simulink model "sampleModel1936_5"  (R2023a)
settings: Solver=VariableStepAuto  StartTime=0.0  StopTime=10.0  RelTol=1e-3
libraries: hdlsllib x7
settings Model: Creator=user1  LastModifiedBy=user1

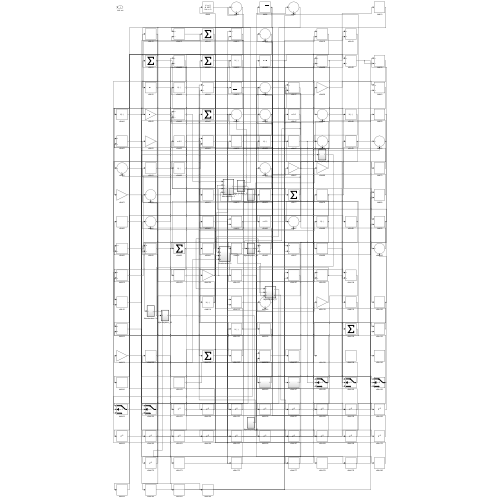
[thumbnail: Simulink's stored preview of the top-level diagram]
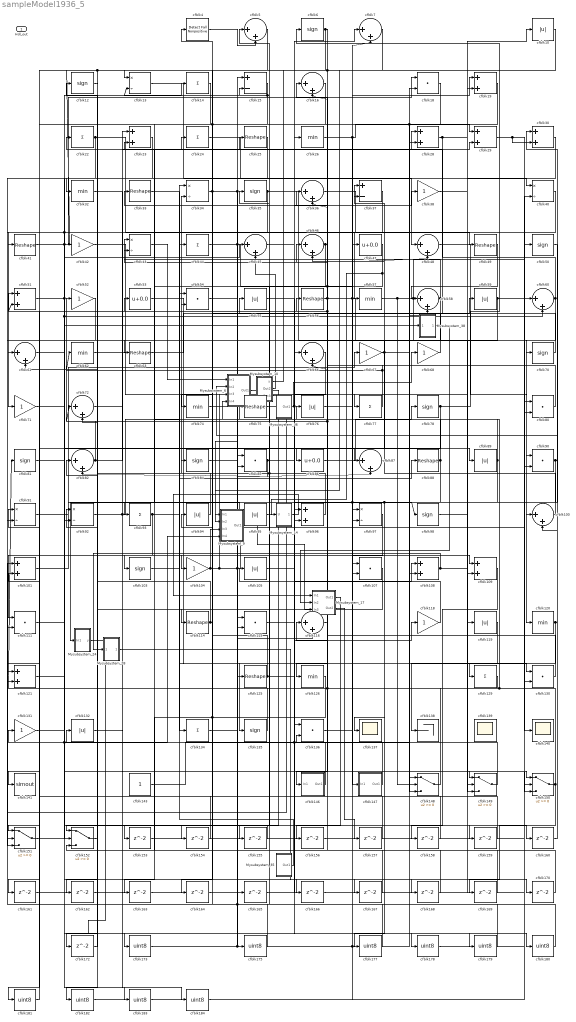
== system sampleModel1936_5 ==
  Mysubsystem_10 : Subsystem  TreatAsAtomicUnit=on  RTWFcnName=Mysubsystem_10
      settings: RTWFcnNameOpts=User specified  RTWFileNameOpts=Use function name
  Mysubsystem_14 : Subsystem  TreatAsAtomicUnit=on  RTWFcnName=Mysubsystem_14
      settings: RTWFcnNameOpts=User specified  RTWFileNameOpts=Use function name
  Mysubsystem_17 : Subsystem  TreatAsAtomicUnit=on  RTWFcnName=Mysubsystem_17
      settings: RTWFcnNameOpts=User specified  RTWFileNameOpts=Use function name
  Mysubsystem_24 : Subsystem  TreatAsAtomicUnit=on  RTWFcnName=Mysubsystem_24
      settings: RTWFcnNameOpts=User specified  RTWFileNameOpts=Use function name
  Mysubsystem_28 : Subsystem  TreatAsAtomicUnit=on  RTWFcnName=Mysubsystem_28
      settings: RTWFcnNameOpts=User specified  RTWFileNameOpts=Use function name
  Mysubsystem_35 : Subsystem  TreatAsAtomicUnit=on  RTWFcnName=Mysubsystem_35
      settings: RTWFcnNameOpts=User specified  RTWFileNameOpts=Use function name
  Mysubsystem_36 : Subsystem  TreatAsAtomicUnit=on  RTWFcnName=Mysubsystem_36
      settings: RTWFcnNameOpts=User specified  RTWFileNameOpts=Use function name
  Mysubsystem_38 : Subsystem  TreatAsAtomicUnit=on  RTWFcnName=Mysubsystem_38
      settings: RTWFcnNameOpts=User specified  RTWFileNameOpts=Use function name
  Mysubsystem_6 : Subsystem  TreatAsAtomicUnit=on  RTWFcnName=Mysubsystem_6
      settings: RTWFcnNameOpts=User specified  RTWFileNameOpts=Use function name
  Mysubsystem_9 : Subsystem  TreatAsAtomicUnit=on  RTWFcnName=Mysubsystem_9
      settings: RTWFcnNameOpts=User specified  RTWFileNameOpts=Use function name
  cfblk{10,55,59,76,89,94..95,105,119,132} (10 alike) : Abs  OutDataTypeStr=uint8  SaturateOnIntegerOverflow=off
  cfblk{5,7,16,36,45..46,48,58,60..61,66,72,82,87,100,116} (16 alike) : Sum  Inputs=|++  OutDataTypeStr=uint8
  cfblk{19,23,28..30,51,96,101,108..109,121} (11 alike) : Sum  OutDataTypeStr=uint8
  cfblk{6,12,35,50,70,78,81,84,98,103,135} (11 alike) : Signum
  cfblk{38,42,52,67..68,71,104,118,131} (9 alike) : Gain  OutDataTypeStr=uint8
  cfblk{18,54,80,85,90,107,111,115,130,136} (10 alike) : DotProduct  OutDataTypeStr=uint8
  cfblk{25,33,41,49,56,63,75,88,114,125} (10 alike) : Reshape
  cfblk{26,32,57,62,74,120,126} (7 alike) : MinMax  OutDataTypeStr=uint8
  cfblk{14,22,24,44,77,93,129,134} (8 alike) : Sum  Inputs=+  OutDataTypeStr=uint8
  cfblk{13,34,40,43,91..92,97} (7 alike) : Product  Inputs=*/  OutDataTypeStr=uint8  RndMeth=Zero  SaturateOnIntegerOverflow=on
  cfblk137 : Scope
  cfblk138 : Terminator
  cfblk139 : Scope
      settings: Floating=on
  cfblk140 : Scope
  cfblk141 : ToWorkspace  VariableName=simout  SaveFormat=Timeseries  SampleTime=-1
  cfblk143 : Constant  OutDataTypeStr=uint8  SampleTime=-1
  cfblk146 : Subsystem
      settings: LibrarySourceBlock=|
      | hdlsllib/Ports &
      | Subsystems/Subsystem
  cfblk147 : Subsystem
      settings: LibrarySourceBlock=|
      | hdlsllib/Ports &
      | Subsystems/Subsystem
  cfblk{148..152} (5 alike) : Switch  OutDataTypeStr=uint8  SaturateOnIntegerOverflow=off  InputSameDT=off
  cfblk15 : Sum  Inputs=+-  OutDataTypeStr=uint8
  cfblk{153..170,172} (19 alike) : Delay  SampleTime=1
  cfblk{173,175,177..184} (10 alike) : DataTypeConversion  OutDataTypeStr=uint8  SaturateOnIntegerOverflow=off  RndMeth=Floor
  cfblk37 : Sum  Inputs=+-  OutDataTypeStr=uint8
  cfblk4 : hdlsllib/Logic and Bit Operations/Detect Fall Nonpositive  vinit=0  OutDataTypeStr=uint8
  cfblk47 : Bias  Bias=0.0  SaturateOnIntegerOverflow=off
  cfblk53 : Bias  Bias=0.0  SaturateOnIntegerOverflow=off
  cfblk86 : Bias  Bias=0.0  SaturateOnIntegerOverflow=off
  Hdl_out : Outport  OutDataTypeStr=uint8
  wires:
  cfblk58/1 -> cfblk43/1, cfblk151/2
  cfblk74/1 -> cfblk77/1
  cfblk49/1 -> cfblk55/1
  cfblk78/1 -> cfblk6/1, cfblk141/1
  cfblk150/1 -> Mysubsystem_6/4(In4), cfblk81/1, cfblk36/1, cfblk169/1
  cfblk82/1 -> cfblk52/1, cfblk25/1
  cfblk97/1 -> cfblk103/1
  cfblk41/1 -> cfblk18/1, cfblk150/1
  cfblk101/1 -> cfblk67/1
  cfblk53/1 -> cfblk135/1
  cfblk88/1 -> Mysubsystem_24/1(In1), cfblk53/1
  cfblk108/1 -> Mysubsystem_28/1(In1), cfblk150/2
  cfblk70/1 -> cfblk4/1
  cfblk130/1 -> cfblk36/2, cfblk51/2, cfblk72/1
  cfblk13/1 -> cfblk97/1
  cfblk48/1 -> cfblk120/1
  cfblk94/1 -> cfblk34/2
  cfblk93/1 -> cfblk111/1, cfblk88/1
  cfblk5/1 -> cfblk121/1
  cfblk118/1 -> cfblk35/1
  cfblk63/1 -> cfblk59/1
  cfblk125/1 -> cfblk24/1, cfblk118/1
  cfblk26/1 -> cfblk29/1, cfblk48/2
  cfblk33/1 -> cfblk89/1
  cfblk126/1 -> cfblk163/1, cfblk164/1
  cfblk46/1 -> cfblk16/1, cfblk155/1
  cfblk35/1 -> cfblk92/2, cfblk111/2, cfblk148/1
  cfblk51/1 -> cfblk14/1, cfblk159/1
  cfblk56/1 -> cfblk90/1, cfblk7/2, cfblk16/2
  cfblk22/1 -> cfblk57/1, cfblk91/2
  cfblk15/1 -> cfblk13/2, cfblk181/1
  cfblk40/1 -> cfblk71/1
  cfblk96/1 -> cfblk15/2, cfblk61/2
  cfblk131/1 -> cfblk180/1
  cfblk76/1 -> cfblk109/1
  cfblk129/1 -> cfblk121/2
  cfblk6/1 -> cfblk126/1, cfblk13/1
  cfblk114/1 -> cfblk84/1, cfblk12/1
  cfblk148/1 -> cfblk76/1, cfblk51/1
  cfblk66/1 -> cfblk96/2
  cfblk34/1 -> cfblk29/2, cfblk87/2, cfblk154/1
  cfblk47/1 -> Mysubsystem_14/1(U), cfblk66/2, cfblk63/1
  cfblk68/1 -> cfblk5/1
  cfblk30/1 -> cfblk104/1
  cfblk147/1(Out1) -> cfblk136/2
  cfblk90/1 -> Mysubsystem_6/2(In2), cfblk177/1
  cfblk80/1 -> cfblk33/1
  cfblk98/1 -> cfblk109/2
  cfblk115/1 -> cfblk108/1
  cfblk24/1 -> cfblk48/1
  cfblk87/1 -> cfblk37/1
  cfblk59/1 -> cfblk60/1, cfblk87/1
  cfblk62/1 -> cfblk134/1
  cfblk28/1 -> cfblk10/1, cfblk58/1
  cfblk89/1 -> cfblk137/1, cfblk115/2, cfblk75/1
  cfblk135/1 -> cfblk82/1
  cfblk60/1 -> cfblk22/1, cfblk70/1
  cfblk95/1 -> cfblk149/1
  cfblk103/1 -> cfblk129/1
  cfblk50/1 -> cfblk100/1
  cfblk120/1 -> cfblk30/1, cfblk149/3
  cfblk71/1 -> cfblk85/2
  cfblk143/1 -> cfblk26/1, cfblk28/2
  cfblk119/1 -> cfblk138/1
  cfblk72/1 -> cfblk23/1
  cfblk23/1 -> cfblk152/2
  cfblk151/1 -> Mysubsystem_38/1(In1), Mysubsystem_9/4(In4)
  cfblk146/1(Out1) -> cfblk91/1
  cfblk29/1 -> cfblk140/1, cfblk30/2
  cfblk136/1 -> cfblk19/1
  cfblk45/1 -> cfblk7/1
  cfblk57/1 -> cfblk119/1, cfblk40/2, cfblk148/2
  cfblk37/1 -> cfblk146/1(In1)
  cfblk67/1 -> cfblk130/1, cfblk37/2
  cfblk84/1 -> cfblk116/2
  cfblk36/1 -> cfblk49/1
  cfblk100/1 -> cfblk46/2
  cfblk14/1 -> cfblk41/1
  cfblk19/1 -> cfblk114/1, cfblk151/1, cfblk108/2
  cfblk85/1 -> cfblk82/2, cfblk28/1
  cfblk44/1 -> Mysubsystem_9/2(In2), cfblk147/1(In1)
  cfblk91/1 -> cfblk95/1
  cfblk4/1 -> cfblk5/2
  cfblk111/1 -> cfblk45/1, cfblk60/2
  cfblk86/1 -> cfblk78/1
  cfblk75/1 -> cfblk98/1, cfblk97/2, cfblk38/1
  cfblk152/1 -> cfblk92/1
  cfblk18/1 -> cfblk61/1
  cfblk92/1 -> cfblk44/1, cfblk150/3
  cfblk38/1 -> cfblk40/1
  cfblk104/1 -> Mysubsystem_9/3(In3), Mysubsystem_6/3(In3), cfblk50/1, cfblk148/3
  cfblk77/1 -> cfblk62/1, cfblk43/2
  cfblk10/1 -> cfblk86/1, cfblk74/1
  cfblk116/1 -> cfblk56/1
  cfblk42/1 -> cfblk149/2
  cfblk16/1 -> cfblk93/1
  cfblk149/1 -> cfblk132/1
  cfblk153/1 -> cfblk90/2
  cfblk154/1 -> cfblk101/2
  cfblk155/1 -> cfblk152/1
  cfblk156/1 -> cfblk46/1
  cfblk157/1 -> cfblk34/1
  cfblk109/1 -> cfblk158/1
  cfblk158/1 -> cfblk15/1
  cfblk159/1 -> cfblk136/1
  cfblk121/1 -> cfblk160/1
  cfblk160/1 -> cfblk100/2
  cfblk52/1 -> cfblk161/1
  cfblk161/1 -> cfblk85/1
  cfblk25/1 -> cfblk162/1
  cfblk163/1 -> cfblk66/1
  cfblk164/1 -> cfblk130/2
  cfblk134/1 -> cfblk165/1
  cfblk165/1 -> cfblk19/2
  cfblk166/1 -> cfblk18/2
  cfblk81/1 -> cfblk167/1
  cfblk167/1 -> cfblk152/3
  cfblk55/1 -> cfblk168/1
  cfblk168/1 -> cfblk116/1
  cfblk169/1 -> cfblk23/2
  cfblk132/1 -> cfblk170/1
  cfblk170/1 -> cfblk96/1
  cfblk12/1 -> cfblk172/1
  cfblk172/1 -> cfblk72/2
  cfblk173/1 -> cfblk58/2, cfblk47/1, cfblk125/1
  cfblk54/1 -> cfblk175/1
  cfblk175/1 -> cfblk94/1
  cfblk177/1 -> cfblk54/2
  cfblk105/1 -> cfblk178/1
  cfblk178/1 -> cfblk80/2
  cfblk32/1 -> cfblk179/1
  cfblk179/1 -> cfblk105/1
  cfblk180/1 -> cfblk115/1, cfblk101/1
  cfblk181/1 -> cfblk131/1
  cfblk107/1 -> cfblk182/1
  cfblk182/1 -> cfblk80/1
  cfblk61/1 -> cfblk183/1
  cfblk183/1 -> cfblk107/1
  cfblk162/1 -> cfblk184/1
  cfblk184/1 -> cfblk107/2
  cfblk43/1 -> Mysubsystem_6/1(In1)
  Mysubsystem_6/1(Out1) -> cfblk153/1
  cfblk7/1 -> Mysubsystem_9/1(In1)
  Mysubsystem_10/1(y) -> cfblk42/1, cfblk32/1
  Mysubsystem_10/2(Out2) -> cfblk45/2
  Mysubsystem_10/3(Out3) -> cfblk151/3
  Mysubsystem_14/1(Out1) -> Mysubsystem_17/1(In1)
  Mysubsystem_9/1(Out1) -> Mysubsystem_17/3(In3)
  Mysubsystem_17/1(Out1) -> cfblk156/1
  Mysubsystem_17/2(Out2) -> cfblk157/1
  Mysubsystem_24/1(y) -> cfblk173/1
  Mysubsystem_28/1(Out1) -> cfblk166/1
  Mysubsystem_35/1(Out1) -> cfblk54/1
  Mysubsystem_36/1(Out1) -> cfblk68/1
  Mysubsystem_38/1(Out1) -> Mysubsystem_17/2(In2)

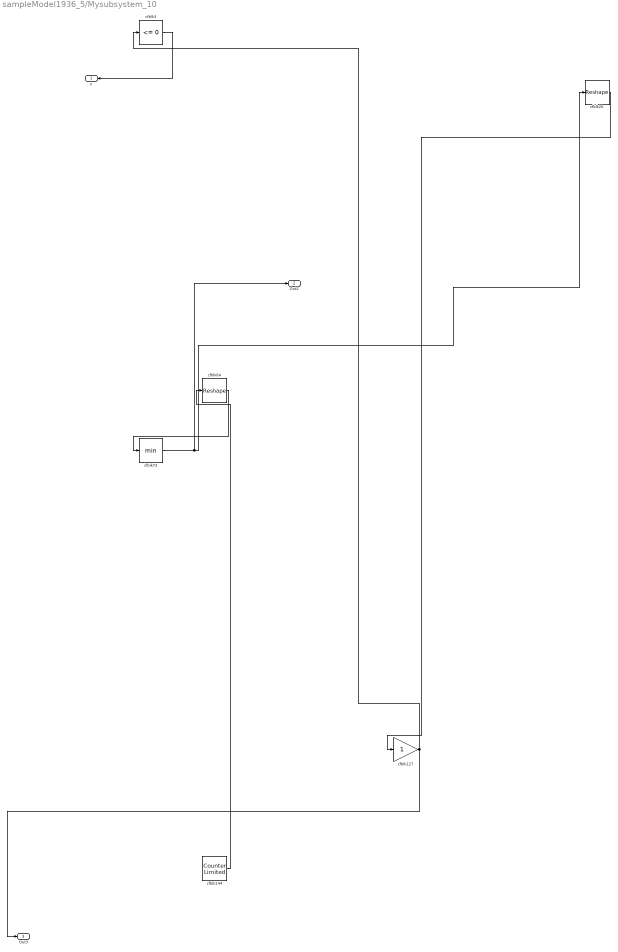
== system sampleModel1936_5/Mysubsystem_10 ==
  cfblk127 : Gain
  cfblk144 : hdlsllib/Sources/Counter Limited  uplimit=7  tsamp=-1
  cfblk20 : Reshape
  cfblk3 : hdlsllib/Logic and Bit Operations/Compare To Zero  relop=<=  OutDataTypeStr=boolean
  cfblk64 : Reshape
  cfblk73 : MinMax
  y : Outport
  Out2 : Outport  Port=2
  Out3 : Outport  Port=3
  wires:
  cfblk64/1 -> cfblk73/1
  cfblk3/1 -> y/1
  cfblk20/1 -> cfblk127/1
  cfblk144/1 -> cfblk64/1
  cfblk127/1 -> Out3/1, cfblk3/1
  cfblk73/1 -> Out2/1, cfblk20/1

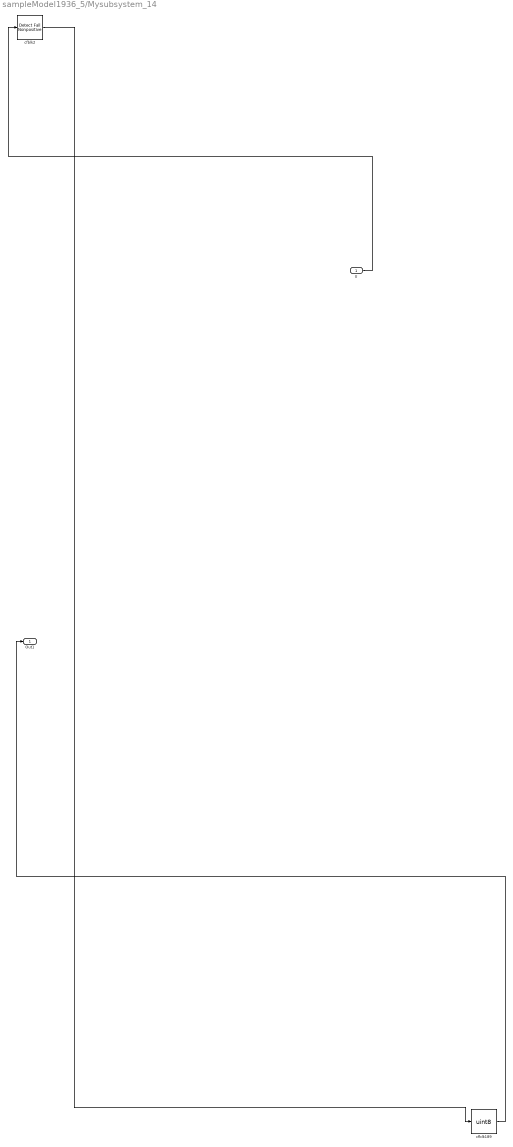
== system sampleModel1936_5/Mysubsystem_14 ==
  U : Inport
  cfblk189 : DataTypeConversion  OutDataTypeStr=uint8  SaturateOnIntegerOverflow=off  RndMeth=Floor
  cfblk2 : hdlsllib/Logic and Bit Operations/Detect Fall Nonpositive  vinit=0  OutDataTypeStr=boolean
  Out1 : Outport
  wires:
  U/1 -> cfblk2/1
  cfblk2/1 -> cfblk189/1
  cfblk189/1 -> Out1/1

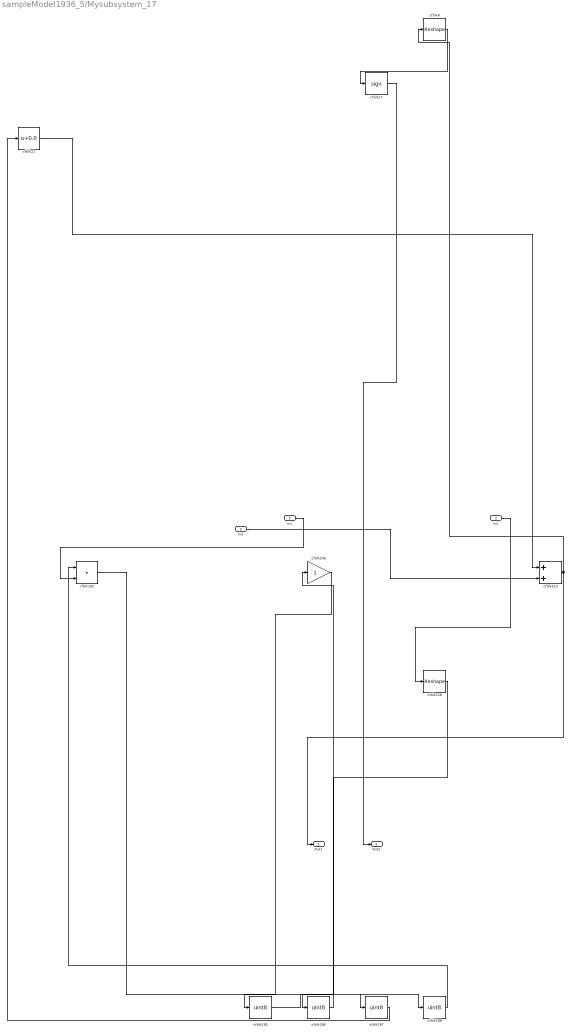
== system sampleModel1936_5/Mysubsystem_17 ==
  In1 : Inport
  In2 : Inport  Port=2
  In3 : Inport  Port=3
  cfblk102 : DotProduct  OutDataTypeStr=Inherit: Inherit via internal rule
  cfblk106 : Gain
  cfblk110 : Sum
  cfblk128 : Reshape
  cfblk17 : Signum
  cfblk{185..188} (4 alike) : DataTypeConversion  OutDataTypeStr=uint8  SaturateOnIntegerOverflow=off  RndMeth=Floor
  cfblk21 : Bias  Bias=0.0  SaturateOnIntegerOverflow=off
  cfblk8 : Reshape
  Out1 : Outport
  Out2 : Outport  Port=2
  wires:
  cfblk21/1 -> cfblk110/1
  cfblk128/1 -> cfblk186/1
  cfblk186/1 -> cfblk106/1
  cfblk187/1 -> cfblk21/1
  In3/1 -> cfblk110/2
  cfblk110/1 -> Out1/1, cfblk8/1
  cfblk185/1 -> cfblk188/1
  cfblk106/1 -> cfblk185/1
  cfblk188/1 -> cfblk102/1
  cfblk102/1 -> cfblk187/1
  cfblk8/1 -> cfblk17/1
  In2/1 -> cfblk128/1
  In1/1 -> cfblk102/2
  cfblk17/1 -> Out2/1

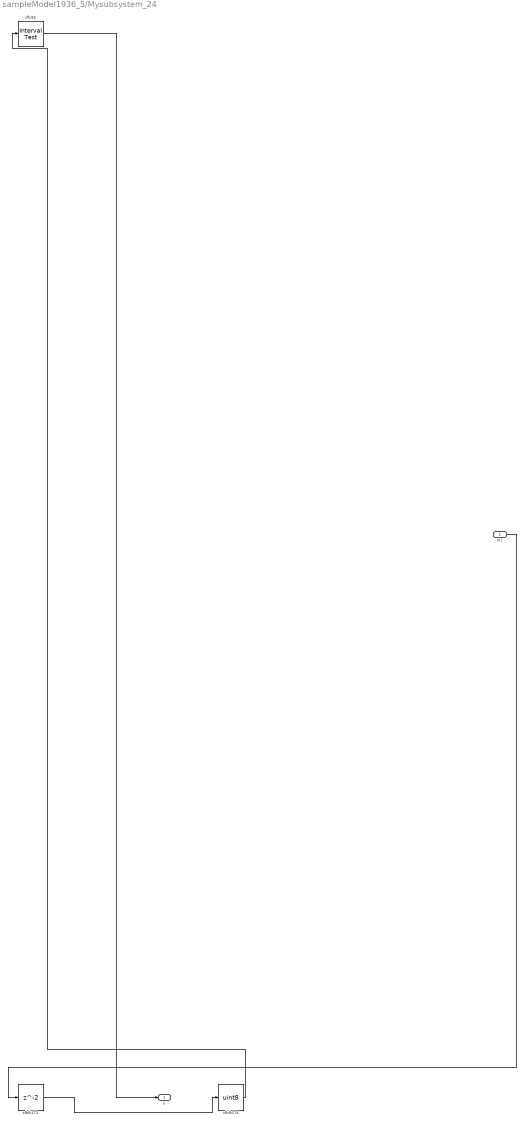
== system sampleModel1936_5/Mysubsystem_24 ==
  In1 : Inport
  cfblk1 : hdlsllib/Logic and Bit Operations/Interval Test  IntervalClosedRight=on  uplimit=0.5  IntervalClosedLeft=on  lowlimit=-0.5  OutDataTypeStr=boolean
  cfblk171 : Delay  SampleTime=1
  cfblk174 : DataTypeConversion  OutDataTypeStr=uint8  SaturateOnIntegerOverflow=off  RndMeth=Floor
  y : Outport
  wires:
  cfblk171/1 -> cfblk174/1
  cfblk174/1 -> cfblk1/1
  In1/1 -> cfblk171/1
  cfblk1/1 -> y/1

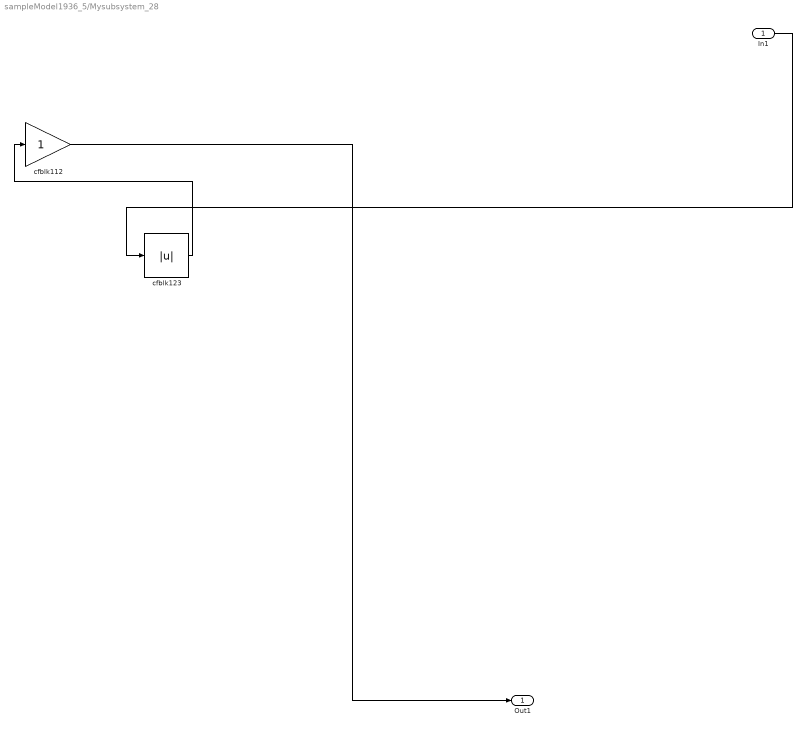
== system sampleModel1936_5/Mysubsystem_28 ==
  In1 : Inport
  cfblk112 : Gain
  cfblk123 : Abs  SaturateOnIntegerOverflow=off
  Out1 : Outport
  wires:
  cfblk123/1 -> cfblk112/1
  In1/1 -> cfblk123/1
  cfblk112/1 -> Out1/1

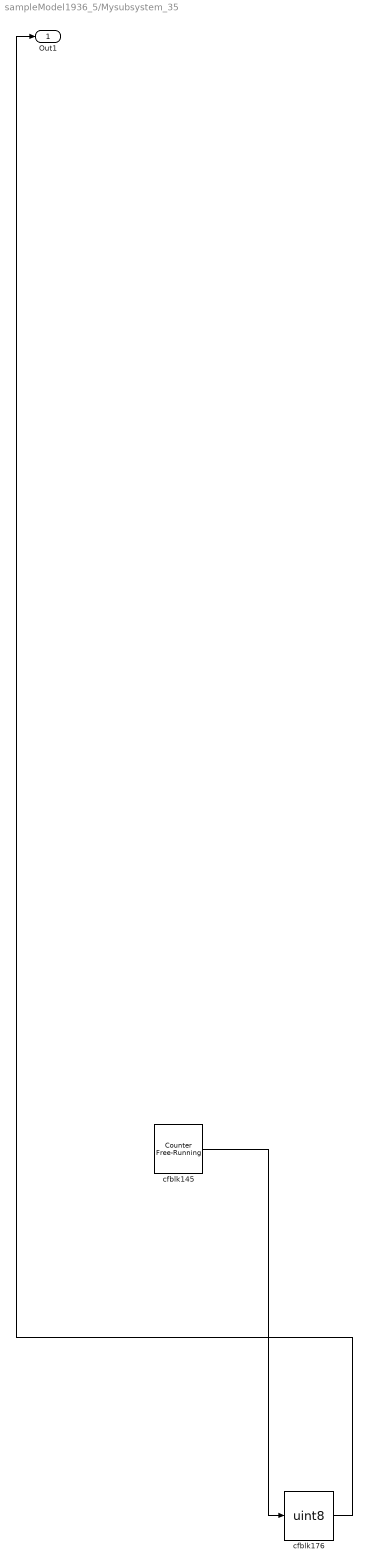
== system sampleModel1936_5/Mysubsystem_35 ==
  cfblk145 : hdlsllib/Sources/Counter Free-Running  NumBits=16  tsamp=-1
  cfblk176 : DataTypeConversion  OutDataTypeStr=uint8  SaturateOnIntegerOverflow=off  RndMeth=Floor
  Out1 : Outport
  wires:
  cfblk145/1 -> cfblk176/1
  cfblk176/1 -> Out1/1

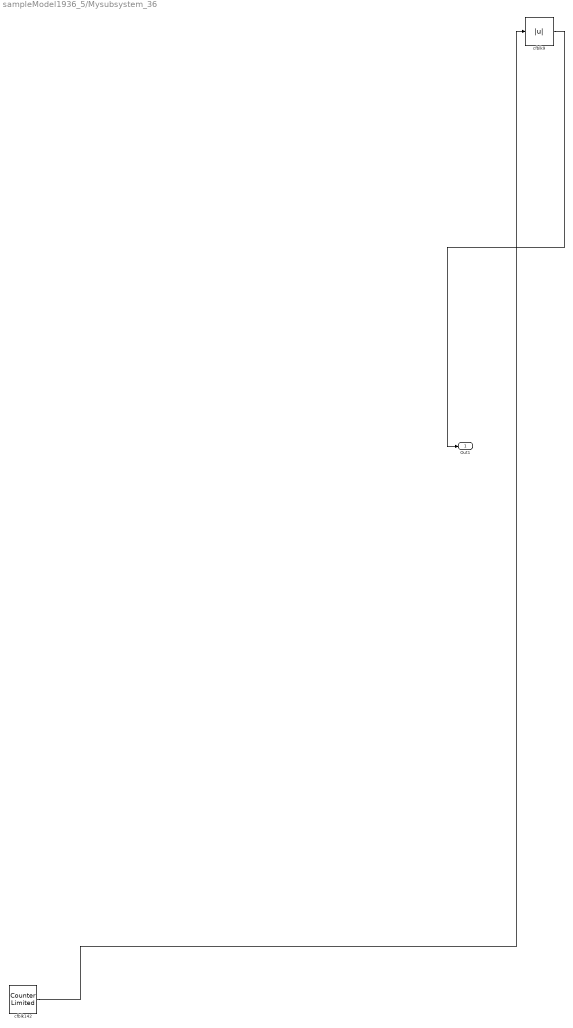
== system sampleModel1936_5/Mysubsystem_36 ==
  cfblk142 : hdlsllib/Sources/Counter Limited  uplimit=7  tsamp=-1
  cfblk9 : Abs  SaturateOnIntegerOverflow=off
  Out1 : Outport
  wires:
  cfblk142/1 -> cfblk9/1
  cfblk9/1 -> Out1/1

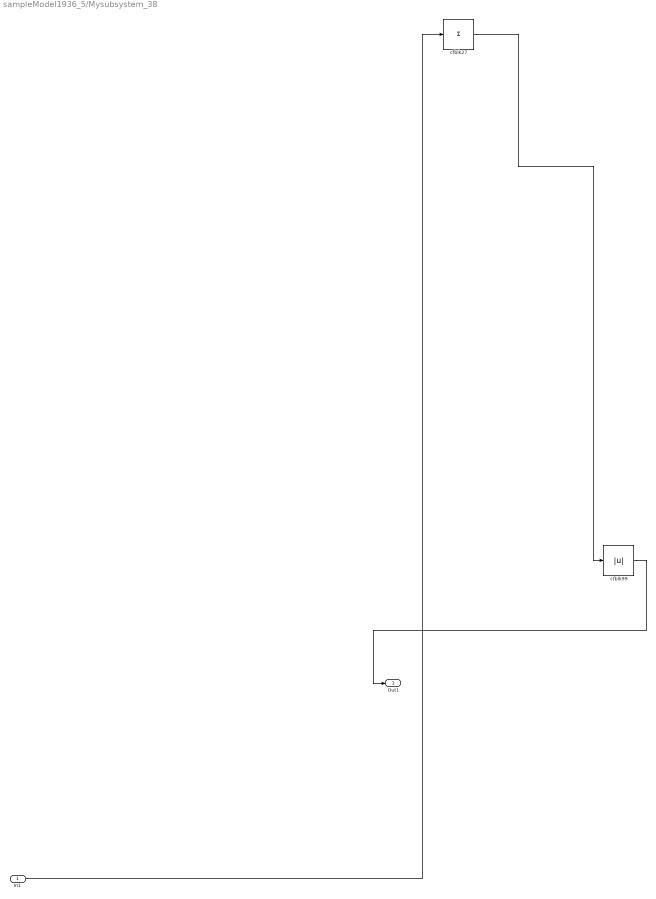
== system sampleModel1936_5/Mysubsystem_38 ==
  In1 : Inport
  cfblk27 : Sum  Inputs=+
  cfblk99 : Abs  SaturateOnIntegerOverflow=off
  Out1 : Outport
  wires:
  cfblk27/1 -> cfblk99/1
  cfblk99/1 -> Out1/1
  In1/1 -> cfblk27/1

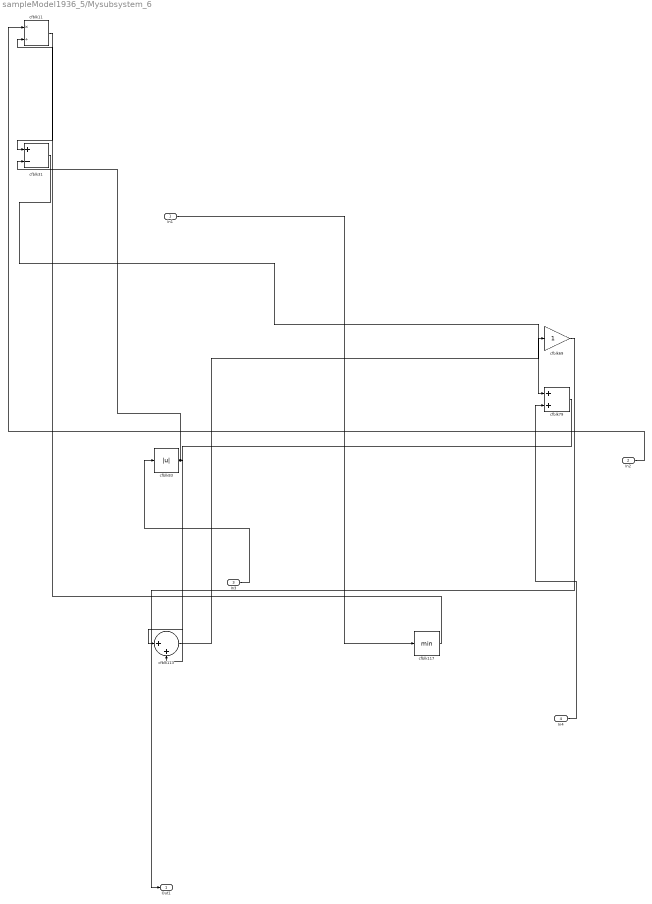
== system sampleModel1936_5/Mysubsystem_6 ==
  In1 : Inport
  In2 : Inport  Port=2
  In3 : Inport  Port=3
  In4 : Inport  Port=4
  cfblk11 : Product  Inputs=*/  RndMeth=Zero  SaturateOnIntegerOverflow=on
  cfblk113 : Sum  Inputs=|++
  cfblk117 : MinMax
  cfblk31 : Sum  Inputs=+-
  cfblk69 : Gain
  cfblk79 : Sum
  cfblk83 : Abs  SaturateOnIntegerOverflow=off
  Out1 : Outport
  wires:
  cfblk69/1 -> Out1/1
  cfblk31/1 -> cfblk79/1
  cfblk117/1 -> cfblk11/2
  In1/1 -> cfblk117/1
  cfblk79/1 -> cfblk113/2
  cfblk83/1 -> cfblk113/1, cfblk31/2
  cfblk11/1 -> cfblk31/1
  cfblk113/1 -> cfblk69/1
  In2/1 -> cfblk11/1
  In3/1 -> cfblk83/1
  In4/1 -> cfblk79/2

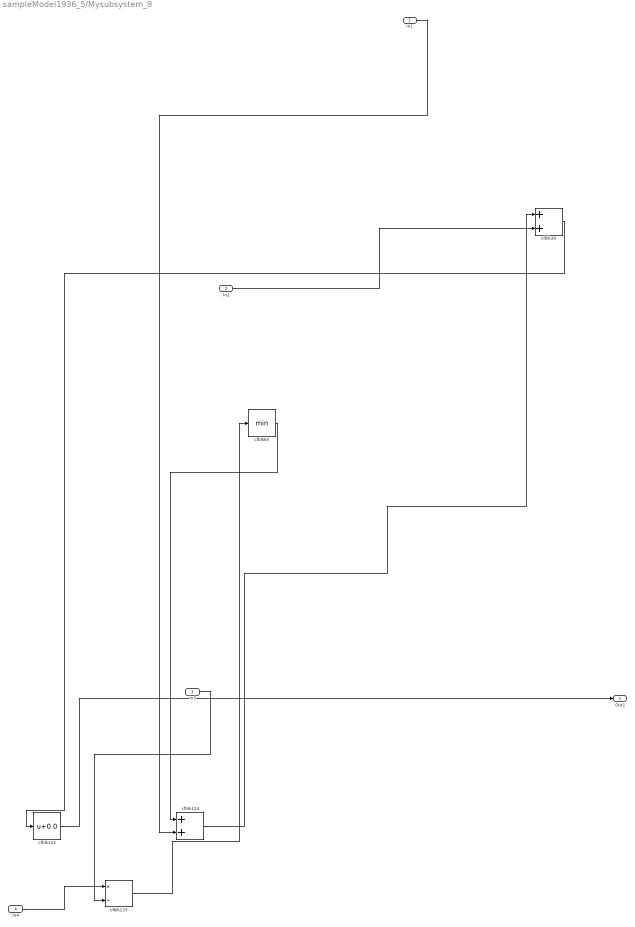
== system sampleModel1936_5/Mysubsystem_9 ==
  In1 : Inport
  In2 : Inport  Port=2
  In3 : Inport  Port=3
  In4 : Inport  Port=4
  cfblk122 : Bias  Bias=0.0  SaturateOnIntegerOverflow=off
  cfblk124 : Sum
  cfblk133 : Product  Inputs=*/  RndMeth=Zero  SaturateOnIntegerOverflow=on
  cfblk39 : Sum
  cfblk65 : MinMax
  Out1 : Outport
  wires:
  cfblk39/1 -> cfblk122/1
  cfblk124/1 -> cfblk39/1
  cfblk133/1 -> cfblk65/1
  cfblk65/1 -> cfblk124/1
  In1/1 -> cfblk124/2
  In4/1 -> cfblk133/1
  cfblk122/1 -> Out1/1
  In2/1 -> cfblk39/2
  In3/1 -> cfblk133/2

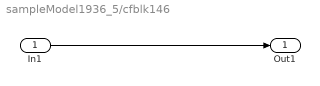
== system sampleModel1936_5/cfblk146 ==
  In1 : Inport
  Out1 : Outport
  wires:
  In1/1 -> Out1/1

== system sampleModel1936_5/cfblk147 ==
  In1 : Inport
  Out1 : Outport
  wires:
  In1/1 -> Out1/1
